simulink model "vocoder_v0"  (R2020a)
settings: Solver=FixedStepDiscrete  StartTime=0.0  StopTime=inf  RelTol=1e-3
libraries: audiosources x2, audiofilters x2, dspsnks4 x1, dspsrcs4 x1
settings Model: Creator=unity  LastModifiedBy=unity
settings SolverCC: AutoInsertRateTranBlk=on
settings DataIOCC: LimitDataPoints=on  SaveOutput=off  SignalLogging=off  SaveTime=off
settings OptimizationCC: LifeSpan=inf
settings DebuggingCC: AlgebraicLoopMsg=error  SingleTaskRateTransMsg=error  AllowSymbolicDim=off  SFUnexpectedBacktrackingDiag=warning  SFNoUnconditionalDefaultTransitionDiag=warning  SFExecutionAtInitializationDiag=none  ArithmeticOperatorsInVariantConditions=warning
settings SFSimCC: SimUseLocalCustomCode=off  CustomCodeUndefinedFunction=UseInterfaceOnly
settings RTWCC: RTWUseLocalCustomCode=off
settings CodeAppCC: StateflowObjectComments=on
settings GRTTargetCC: TargetLangStandard=C89/C90 (ANSI)
settings ConfigComp: CovMetricSettings=dw  CovHtmlReporting=on  CovSaveCumulativeToWorkspaceVar=on  CovSaveSingleToWorkspaceVar=on  CovExternalEMLEnable=off  CovSFcnEnable=off

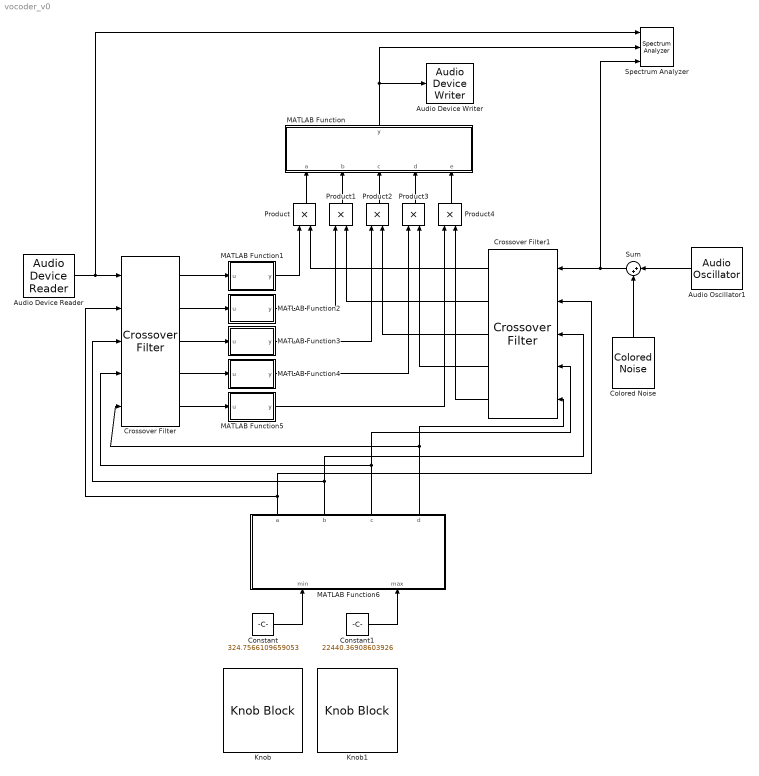
== system vocoder_v0 ==
  Audio Device Reader : audiosources/Audio Device Reader  Driver=DirectSound  Device=Default  SampleRate=44100  NumChannels=1  SamplesPerFrame=1024  BitDepth=16-bit integer  NumBuffers=10  DefaultInputChannelMapping=on  InputChannelMapping=1:2  OutputNumOverrunSamples=off  OutputDataType=double  DriverIdx=1  DeviceWarnFlag=''
      settings: SourceProductBaseCode=AU
  Audio Device Writer : dspsnks4/Audio Device Writer  Driver=DirectSound  Device=Default  InheritSampleRate=on  SampleRate=44100  BitDepth=16-bit integer  BufferSize=4096  NumBuffers=10  DefaultOutputChannelMapping=on  OutputChannelMapping=1:2  OutputNumUnderrunSamples=off  DriverIdx=1  DeviceWarnFlag=''
  Audio Oscillator1 : audiosources/Audio Oscillator  FrequencyPort=off  Frequency=100  AmplitudePort=off  Amplitude=1  DCOffsetPort=off  PhaseOffset=0  DCOffset=0  WidthPort=off  Width=1  DutyCyclePort=off  DutyCycle=0.5  SampsPerFrame=1024  Fs=44100  OutputDataType=double  SimulateUsing=Code generation
      settings: SourceProductBaseCode=AU  SignalType=sawtooth
  Colored Noise : dspsrcs4/Colored Noise  Color=white  InverseFrequencyPower=1  BoundedOutput=off  NumChannels=1  OutputDataType=double  SamplesPerFrame=1024  SampleTime=1  RandomStream=mt19937ar with seed  Seed=67  SimulateUsing=Code generation
      settings: SourceProductBaseCode=DS
  Constant : Constant  Value=324.7566109659053
  Constant1 : Constant  Value=22440.36908603926
  Crossover Filter : audiofilters/Crossover Filter  NCrossovers=4  Crossover1Port=on  Crossover1=500  Order1Port=off  Order1=5  Crossover2Port=on  Crossover2=600  Order2Port=off  Order2=5  Crossover3Port=on  Crossover3=700  Order3Port=off  Order3=5  Crossover4Port=on  Crossover4=800  Order4Port=off  Order4=5  InheritSampleRate=off  SampleRate=44100  SimulateUsing=Code generation
      settings: SourceProductBaseCode=AU
  Crossover Filter1 : audiofilters/Crossover Filter  NCrossovers=4  Crossover1Port=on  Crossover1=500  Order1Port=off  Order1=5  Crossover2Port=on  Crossover2=600  Order2Port=off  Order2=5  Crossover3Port=on  Crossover3=700  Order3Port=off  Order3=5  Crossover4Port=on  Crossover4=800  Order4Port=off  Order4=5  InheritSampleRate=off  SampleRate=44100  SimulateUsing=Code generation
      settings: SourceProductBaseCode=AU
  Knob : KnobBlock  ScaleMin=200  ScaleMax=20000  ScaleType=Log
  Knob1 : KnobBlock  ScaleMin=20  ScaleMax=20000  ScaleType=Log
  MATLAB Function : MATLAB Function  TreatAsAtomicUnit=on
  MATLAB Function1 : MATLAB Function  TreatAsAtomicUnit=on
  MATLAB Function2 : MATLAB Function  TreatAsAtomicUnit=on
  MATLAB Function3 : MATLAB Function  TreatAsAtomicUnit=on
  MATLAB Function4 : MATLAB Function  TreatAsAtomicUnit=on
  MATLAB Function5 : MATLAB Function  TreatAsAtomicUnit=on
  MATLAB Function6 : MATLAB Function  TreatAsAtomicUnit=on
  Product{,1..4} (5 alike) : Product
  Spectrum Analyzer : SpectrumAnalyzer  NumInputPorts=3
  Sum : Sum  Inputs=|++
  wires:
  Audio Device Reader/1 -> Spectrum Analyzer/1, Crossover Filter/1
  Crossover Filter/1 -> MATLAB Function1/1(u)
  Crossover Filter/2 -> MATLAB Function2/1(u)
  Crossover Filter/3 -> MATLAB Function3/1(u)
  Crossover Filter/4 -> MATLAB Function4/1(u)
  Crossover Filter/5 -> MATLAB Function5/1(u)
  MATLAB Function1/1(y) -> Product/1
  Crossover Filter1/1 -> Product/2
  Crossover Filter1/2 -> Product1/2
  Crossover Filter1/3 -> Product2/2
  Crossover Filter1/4 -> Product3/2
  Crossover Filter1/5 -> Product4/2
  Product/1 -> MATLAB Function/1(a)
  Product1/1 -> MATLAB Function/2(b)
  Product2/1 -> MATLAB Function/3(c)
  Product3/1 -> MATLAB Function/4(d)
  Product4/1 -> MATLAB Function/5(e)
  MATLAB Function/1(y) -> Spectrum Analyzer/2, Audio Device Writer/1
  MATLAB Function2/1(y) -> Product1/1
  MATLAB Function3/1(y) -> Product2/1
  MATLAB Function4/1(y) -> Product3/1
  MATLAB Function5/1(y) -> Product4/1
  Audio Oscillator1/1 -> Sum/1
  Sum/1 -> Spectrum Analyzer/3, Crossover Filter1/1
  Colored Noise/1 -> Sum/2
  MATLAB Function6/4(d) -> Crossover Filter1/5, Crossover Filter/5
  MATLAB Function6/3(c) -> Crossover Filter1/4, Crossover Filter/4
  MATLAB Function6/2(b) -> Crossover Filter1/3, Crossover Filter/3
  MATLAB Function6/1(a) -> Crossover Filter1/2, Crossover Filter/2
  Constant/1 -> MATLAB Function6/1(min)
  Constant1/1 -> MATLAB Function6/2(max)

== matlab function vocoder_v0/MATLAB Function1 ==
  data: u input; y output
function y = fcn(u)

y = sum(u.*u);

== matlab function vocoder_v0/MATLAB Function ==
  data: a input; y output; b input; c input; d input; e input
function y = fcn(a,b,c,d,e)

y = a+b+c+d+e;

== matlab function vocoder_v0/MATLAB Function2 ==
  data: u input; y output
function y = fcn(u)

y = sum(u.*u);

== matlab function vocoder_v0/MATLAB Function3 ==
  data: u input; y output
function y = fcn(u)

y = sum(u.*u);

== matlab function vocoder_v0/MATLAB Function4 ==
  data: u input; y output
function y = fcn(u)

y = sum(u.*u);

== matlab function vocoder_v0/MATLAB Function5 ==
  data: u input; y output
function y = fcn(u)

y = sum(u.*u);

== matlab function vocoder_v0/MATLAB Function6 ==
  data: min input; a output; max input; b output; c output; d output
function [a,b,c,d] = fcn(min,max)
    range = max/min;
    a = min*range^(0/3);
    b = min*range^(1/3);
    c = min*range^(2/3);
    d = min*range^(3/3);
